simulink model "q22"  (R2024a)
settings: Solver=VariableStepAuto  StartTime=0.0  StopTime=10.0  RelTol=1e-3
settings Model: Creator=kiani  LastModifiedBy=kiani

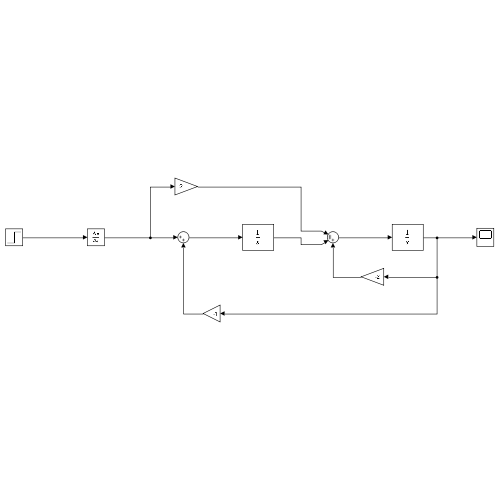
[thumbnail: Simulink's stored preview of the top-level diagram]
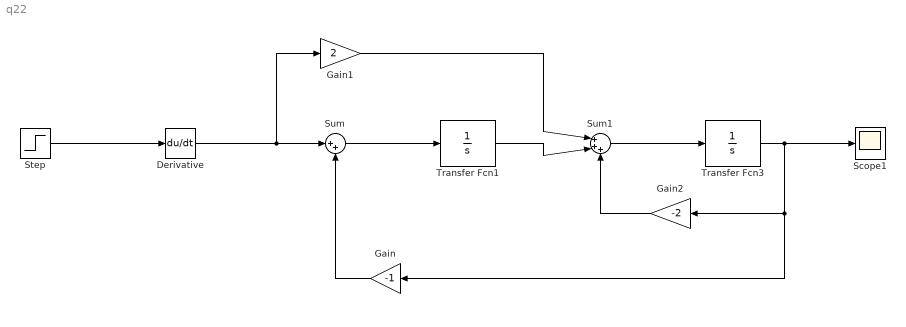
== system q22 ==
  Derivative : Derivative
  Gain : Gain  Gain=-1
  Gain1 : Gain  Gain=2
  Gain2 : Gain  Gain=-2
  Scope1 : Scope
  Step : Step  Time=0.001  After=21.4285712  SampleTime=0
  Sum : Sum  Inputs=|++
  Sum1 : Sum  Inputs=|+++
  Transfer Fcn1 : TransferFcn  Numerator=[0 1]  Denominator="[ 1  0]"
  Transfer Fcn3 : TransferFcn  Numerator=[0 1]  Denominator="[ 1  0]"
  wires:
  Transfer Fcn1/1 -> Sum1/2
  Transfer Fcn3/1 -> Scope1/1, Gain/1, Gain2/1
  Sum1/1 -> Transfer Fcn3/1
  Sum/1 -> Transfer Fcn1/1
  Gain/1 -> Sum/2
  Derivative/1 -> Gain1/1, Sum/1
  Gain2/1 -> Sum1/3
  Step/1 -> Derivative/1
  Gain1/1 -> Sum1/1
